simulink model "Cart_Pendulum_Linearised_a_n9945008"  (R2018b)
settings: Solver=VariableStepAuto  StartTime=0.0  StopTime=10.0  RelTol=1e-3
values from neighbouring files (symbols this model uses):
  g = 9.81    [CP_SFC_Lin_a_MainFile_n9945008.m]    (also in CP_SFC_Lin_b_MainFile_n9945008.m; MainFile_n9945008.m)
  l = 0.2    [CP_SFC_Lin_a_MainFile_n9945008.m]    (also in CP_SFC_Lin_b_MainFile_n9945008.m; Cart_Pendulum_Animation.m; MainFile_n9945008.m)
  m = 0.15    [CP_SFC_Lin_a_MainFile_n9945008.m]    (also in CP_SFC_Lin_b_MainFile_n9945008.m; MainFile_n9945008.m; sim_msd_diff_solvers.m = 1)
  Mc = 0.4    [CP_SFC_Lin_a_MainFile_n9945008.m]    (also in CP_SFC_Lin_b_MainFile_n9945008.m; MainFile_n9945008.m)
settings Model: Creator=Cody  LastModifiedBy=Cody

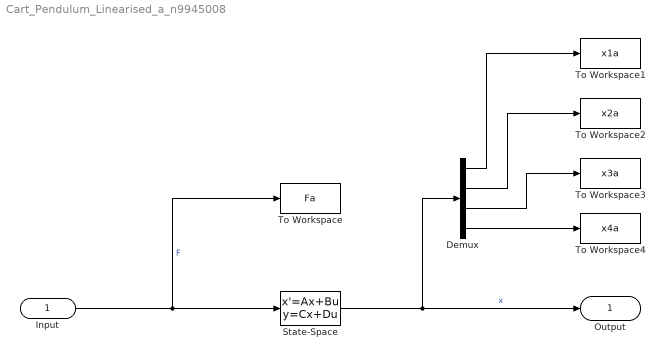
== system Cart_Pendulum_Linearised_a_n9945008 ==
  Input : Inport
  Demux : Demux
  State-Space : StateSpace  A=[0,0,1,0;0,0,0,1;0,-(g*m)/Mc,0,0;0,(g*(Mc+m))/l*Mc,0,0]  B=[0;0;1/Mc;1/l*Mc]  C=eye(4)  D=zeros(4,1)  InitialCondition=0
  To Workspace : ToWorkspace  VariableName=Fa  SaveFormat=Timeseries  SampleTime=-1
  To Workspace1 : ToWorkspace  VariableName=x1a  SaveFormat=Timeseries  SampleTime=-1
  To Workspace2 : ToWorkspace  VariableName=x2a  SaveFormat=Timeseries  SampleTime=-1
  To Workspace3 : ToWorkspace  VariableName=x3a  SaveFormat=Timeseries  SampleTime=-1
  To Workspace4 : ToWorkspace  VariableName=x4a  SaveFormat=Timeseries  SampleTime=-1
  Output : Outport
  wires:
  Input/1 -> To Workspace/1, State-Space/1  "F"
  State-Space/1 -> Demux/1, Output/1  "x"
  Demux/1 -> To Workspace1/1
  Demux/2 -> To Workspace2/1
  Demux/3 -> To Workspace3/1
  Demux/4 -> To Workspace4/1
